simulink model "dut_shape_mod"  (R2020b)
settings: Solver=FixedStepDiscrete  StartTime=0.0  StopTime=10.0  RelTol=1e-3
undefined symbols (not defined in the file or in its folder): srrc_trans_coeffs
libraries: commdigbbndpm3 x1, commrandsrc3 x1
settings Model: DataTypeOverride=Off  Creator=wardo  LastModifiedBy=wardo
settings DataIOCC: LimitDataPoints=on  SaveOutput=off  SaveTime=off
settings OptimizationCC: BlockReduction=off  ConditionallyExecuteInputs=off  DefaultParameterBehavior=Inlined  LifeSpan=inf
settings DebuggingCC: AlgebraicLoopMsg=error  SingleTaskRateTransMsg=error  AllowSymbolicDim=off  StrictBusMsg=ErrorOnBusTreatedAsVector  SFUnexpectedBacktrackingDiag=warning  SFNoUnconditionalDefaultTransitionDiag=warning  SFExecutionAtInitializationDiag=none  ArithmeticOperatorsInVariantConditions=warning
settings HardwareCC: ProdBitPerPointer=32  ProdBitPerSizeT=32  ProdBitPerPtrDiffT=32  ProdLargestAtomicFloat=None  ProdIntDivRoundTo=Undefined  ProdEndianess=Unspecified  ProdWordSize=32  ProdHWDeviceType=ASIC/FPGA->ASIC/FPGA  ProdEqTarget=off
settings SFSimCC: SimUseLocalCustomCode=off  CustomCodeUndefinedFunction=UseInterfaceOnly
settings RTWCC: RTWUseLocalCustomCode=off
settings CodeAppCC: StateflowObjectComments=on
settings GRTTargetCC: TargetLangStandard=C89/C90 (ANSI)
settings ConfigComp: CovScope=ReferencedModels  CovMetricSettings=dw  CovSaveCumulativeToWorkspaceVar=on  CovSaveSingleToWorkspaceVar=on  CovExternalEMLEnable=off  CovSFcnEnable=off

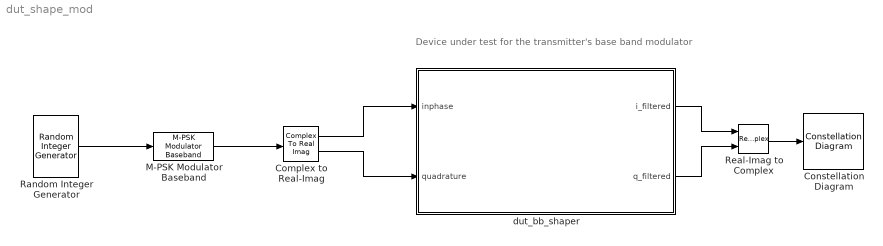
== system dut_shape_mod ==
  note: Device under test for the transmitter's base band modulator
  Complex to Real-Imag : ComplexToRealImag
  Constellation Diagram : ConstellationDiagram
  M-PSK Modulator Baseband : commdigbbndpm3/M-PSK Modulator Baseband  M=8  InType=Bit  Enc=Gray  Mapping=[0:7]  Ph=0  outDtype=Fixed-point  outWordLen=18  outUDDataType=sfix(16)  outFracLenMode=User-defined  outFracLen=14  outDataTypeStr=fixdt(1,18,14)  outLastDataTypeStr=fixdt(1,18,14)
      settings: SourceProductName=Communications Toolbox
  Random Integer Generator : commrandsrc3/Random Integer Generator  SetSize=2  SeedSource=Auto  Seed=0  SampleTime=1  SamplesPerFrame=64800  OutputDataType=double  SimulateUsing=Interpreted execution
  Real-Imag to Complex : RealImagToComplex
  dut_bb_shaper : Subsystem
  wires:
  Complex to Real-Imag/1 -> dut_bb_shaper/1(inphase)
  Complex to Real-Imag/2 -> dut_bb_shaper/2(quadrature)
  M-PSK Modulator Baseband/1 -> Complex to Real-Imag/1
  Random Integer Generator/1 -> M-PSK Modulator Baseband/1
  Real-Imag to Complex/1 -> Constellation Diagram/1
  dut_bb_shaper/1(i_filtered) -> Real-Imag to Complex/1
  dut_bb_shaper/2(q_filtered) -> Real-Imag to Complex/2

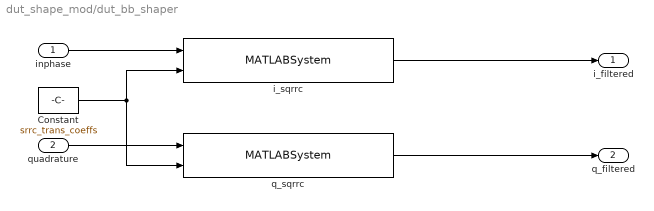
== system dut_shape_mod/dut_bb_shaper ==
  inphase : Inport
  quadrature : Inport  Port=2
  Constant : Constant  Value=srrc_trans_coeffs  OutDataTypeStr=fixdt(1,16)  SampleTime=-1
  i_sqrrc : MATLABSystem  System=transmit_srrc_filter  l=21600  interpolation_factor=8  SimulateUsing=Code generation
      mask Type: transmit_srrc_filter
      mask Display:
      | disp('transmit_srrc_filter');
      | port_label('input',1,'x');
      | port_label('input',2,'coefficients');
      | port_label('output',1,'x_filtered');
  q_sqrrc : MATLABSystem  System=transmit_srrc_filter  l=21600  interpolation_factor=8  SimulateUsing=Code generation
      mask Type: transmit_srrc_filter
      mask Display:
      | disp('transmit_srrc_filter');
      | port_label('input',1,'x');
      | port_label('input',2,'coefficients');
      | port_label('output',1,'x_filtered');
  i_filtered : Outport  VectorParamsAs1DForOutWhenUnconnected=off
  q_filtered : Outport  Port=2  VectorParamsAs1DForOutWhenUnconnected=off
  wires:
  i_sqrrc/1 -> i_filtered/1
  q_sqrrc/1 -> q_filtered/1
  inphase/1 -> i_sqrrc/1
  quadrature/1 -> q_sqrrc/1
  Constant/1 -> q_sqrrc/2, i_sqrrc/2
